simulink model "VCM20_TCon"  (R2021b)
settings: Solver=ode1  StartTime=0.0  StopTime=Inf  FixedStep=0.001  RelTol=1e-3
PostLoadFcn:
  | , if any(exist('dsrtsu_mdlpostloadfcn', 'file') ~= 0), dsrtsu_mdlpostloadfcn('Execute', bdroot); end,
values from neighbouring files (symbols this model uses):
  gear_f = 14.45    [VehicleParamsFEM20_Gear17.m]
  Rwf = 18*(25.4/1000)/2    (= 0.2286)    [VehicleParamsFEM20_Gear17.m]
libraries: rtican x62, dspstat3 x9, simulink x8, rti1401lib_dio_type4 x4, rti1401lib_adc_type4 x4
(part 12 of 12)

== system VCM20_TCon/CAN to EVO4S/relay to EVO4s ==
  from relay board : Inport
  Bus Selector : BusSelector  OutputSignals=AMS_shutdownsig,BSPD_shutdownsig,IMD_shutdownsig
  Data Type Conversion1 : DataTypeConversion
  Data Type Conversion10 : DataTypeConversion
  Data Type Conversion2 : DataTypeConversion
  to EVO4s 704 : rtican/RTICAN Transmit (TX)   Reserved1=[]  Reserved2=[]  Reserved3=[]  Reserved4=[]  SfcnMessage=[]  Msg_Struct=[]  BoardTypeNo=[]  BoardNo=[]  ChannelNo=[]  Parameters=[]  DialogFcn=[]  UnitName=[]  Revision=[]  UnitValues=[]  DSProperties=struct('RTI',struct('Version',uint32(5),'BlockType',struct('isSLSource',uint8(1),'isSLSink',uint8(1),'isHWSource',uint8(0),'isHWSink',uint8(0),'isSetup',uint8(0),'isInline',uint8(1),'isNonInline',uint8(0),'isInterrupt',uint8(0),'isChannelwise',uint8(0)),'IOBoardType','RTICAN','UnitType','MESSAGE','Identifier','TX','DialogType','MSVC','BlockSet','RTICAN','SlaveProcessor','CAN'))  RTIBlockInterface=struct('InputPortsWidth',int32([1 1 1]),'InputPortsActive',[1 1 1],'InputPortsName',{{'AMS_shutdownsig','BSPD_shutdownsig','IMD_shutdownsig'}},'InputPortsDataType',{{'SS_DOUBLE','SS_DOUBLE','SS_DOUBLE'}},'OutputPortsWidth',int32(0),'OutputPortsActive',0,'OutputPortsName',{{''}},'DialogFcn','rtican_message_interface_gui','BlockDisplay',{{'','center'}},'IconTransparency','on','InitLevel',3,'BlockName',struct('Token',{{'CAN_TYPE','_TX_M','_C'}},'BlockParam',{{'BoardTypeNo','BoardNo','ChannelNo'}}),'SampleTime',{{-1}},'TriggerPort',{{'none'}},'EnablePort',{{'none'}})  RTIBlockParameters=struct('BoardTypeNo',{{1,'OFF',[]}},'BoardNo',{{1,'ON',[1 16]}},'ChannelNo',{{2,'ON',[1 2]}},'Parameters',{{struct('DataFileSupport',struct('DataFileSelectedMaster',0,'DataFileSelectedLocal',0,'DataFileName',['<no datafile support>|'],'DataFileDate','','SelectedFile',['<no file selected>']),'Options',struct('StatusSelected',0,'TimeSelected',0,'DeltaTimeSelected',0,'DelayTimeSelected',0,'DelayTimeTXCommandSelected',0,'EncodeSetUnusedBitsToOne',0,'EnableMsgLoopback',0,'TriggerPort',struct('Selected',0,'TriggerType',0),'EnablePortSelected',0,'SignalOnPortnameSelected',1,'UserCoding',struct('Selected',0,'InterfaceFile','UserEncodingFile','FcnName','UserEncodeFcn','InportSelected',0,'InportWidth',1,'OutportSelected',0,'OutportWidth',1),'TerminationMsg',struct('Selected',0,'Byte0_7','0'),'InitialMsg',struct('Selected',0,'Byte0_7','0')),'Message',struct('MsgOnBlocknameSelected',0,'MsgName','EVO4s005','MsgIdFormat',0,'MsgId',1796,'MsgLength',8,'NumSignals',3,'SampleTime',-1,'StartTime',struct('Selected',0,'Value',0),'AutoRepeatTime',struct('Selected',0,'Value',0.1),'Timeout',struct('Selected',0,'Value',0.1),'DelayTime',struct('Selected',0,'Value',0.1),'Signal',struct('SgnName',{'AMS_shutdownsig','BSPD_shutdownsig','IMD_shutdownsig'},'SgnStartBit',{0,1,2},'SgnLength',{1,1,1},'SgnType',{0,0,0},'ModeValue',{-1,-1,-1},'DataType',{1,1,1},'ByteLayout',{1,1,1},'Factor',{1,1,1},'Offset',{0,0,0},'SgnComment',{{''},{''},{''}},'SgnUnit',{'','',''},'Min',{0,0,0},'Max',{0,0,0},'SLDataType',{'SS_DOUBLE','SS_DOUBLE','SS_DOUBLE'}),'MsgIdNumFormat',1,'MsgComment',{{''}}),'Version',1.2,'general',struct('isFromLib',0)),'OFF',[]}},'GroupId',{{struct('Group',{{'RTICAN'}},'No',2,'Behavior',{{'NAMECHANGE'}},'BlockType',{{'SINK'}},'NameChangeFlag',0),'OFF',[]}},'SFcnRTICANMessage',{{struct('MsgType','TX','SFcnPortType','Scalar','MsgName','EVO4s005','MsgIdFormat','STD','MsgId',1796,'MsgLength',8,'NumSignals',3,'SampleTime',-1,'StartTime',struct('Selected','no','Value',0),'AutoRepeatTime',struct('Selected','no','Value',0.1),'Timeout',struct('Selected','no','Value',0.1),'Signal',struct('SgnName',{'AMS_shutdownsig','BSPD_shutdownsig','IMD_shutdownsig'},'SgnStartBit',{0,1,2},'SgnLength',{1,1,1},'SgnType',{'standard','standard','standard'},'ModeValue',{-1,-1,-1},'DataType',{['signed int'],['signed int'],['signed int']},'ByteLayout',{['big endian'],['big endian'],['big endian']},'Factor',{1,1,1},'Offset',{0,0,0},'SLDataType',{'SS_DOUBLE','SS_DOUBLE','SS_DOUBLE'}),'StatusSelected','no','TimeSelected','no','DeltaTimeSelected','no','DelayTimeSelected','no','DelayTimeTXCommandSelected','no','EncodeSetUnusedBitsToOne','no','EnableMsgLoopback','no','TriggerPort',struct('Selected','no','TriggerType',0),'EnablePortSelected','no','UserCoding',struct('Selected','no','InterfaceFile','UserEncodingFile','FcnName','UserEncodeFcn','InportSelected','no','InportWidth',1,'OutportSelected','no','OutportWidth',1),'TerminationMsg',struct('Selected','no','Byte0','0x00','Byte1','0x00','Byte2','0x00','Byte3','0x00','Byte4','0x00','Byte5','0x00','Byte6','0x00','Byte7','0x00'),'InitialMsg',struct('Selected','no','Byte0','0x00','Byte1','0x00','Byte2','0x00','Byte3','0x00','Byte4','0x00','Byte5','0x00','Byte6','0x00','Byte7','0x00'),'BoardType','DS1','BoardNo',1,'ControllerNo',2),'OFF',[]}},'TLCFileName',{{'rtican_tx_message','OFF',[]}})  RTISFcnParameters=struct('SFcnRTICANMessage','struct','TLCFileName','char')  RTIBlockParaDefault=struct('BoardTypeNo',4302,'BoardNo',1,'ChannelNo',1,'Parameters',struct('DataFileSupport',struct('DataFileSelectedMaster',0,'DataFileSelectedLocal',0,'DataFileName','','DataFileDate','','SelectedFile',['<no file selected>']),'Options',struct('StatusSelected',1,'TimeSelected',1,'DeltaTimeSelected',1,'DelayTimeSelected',1,'DelayTimeTXCommandSelected',0,'EncodeSetUnusedBitsToOne',0,'EnableMsgLoopback',0,'TriggerPort',struct('Selected',0,'TriggerType','rising'),'EnablePortSelected',0,'SignalOnPortnameSelected',1,'UserCoding',struct('Selected',0,'InterfaceFile','UserEncodingFile','FcnName','UserEncodeFcn','InportSelected',0,'InportWidth',1,'OutportSelected',0,'OutportWidth',1),'TerminationMsg',struct('Selected',0,'Byte0_7','0'),'InitialMsg',struct('Selected',0,'Byte0_7','0')),'Message',struct('MsgOnBlocknameSelected',0,'MsgName',['TX Message'],'MsgIdFormat',0,'MsgId',100,'MsgLength',8,'NumSignals',1,'SampleTime',-1,'StartTime',struct('Selected',0,'Value',0),'AutoRepeatTime',struct('Selected',0,'Value',0.1),'Timeout',struct('Selected',0,'Value',0.1),'DelayTime',struct('Selected',0,'Value',0.1),'Signal',struct('SgnName',['TX signal'],'SgnStartBit',0,'SgnLength',8,'SgnType',0,'ModeValue',-1,'DataType',0,'SLDataType','SS_DOUBLE','ByteLayout',0,'Factor',1,'Offset',0,'Min',0,'Max',255,'SgnComment',{{}},'SgnUnit',''),'MsgIdNumFormat',0,'MsgComment',{{''}}),'Version',1.2,'general',struct('isFromLib',1)),'GroupId',struct('Group',{{'RTICAN'}},'No',1,'Behavior',{{'NAMECHANGE'}},'BlockType',{{'SINK'}},'NameChangeFlag',0),'SFcnRTICANMessage',struct('MsgType','TX','MsgName',['TX Message'],'MsgIdFormat','STD','MsgId',100,'MsgLength',2,'NumSignals',1,'SampleTime',-1,'StartTime',struct('Selected','no','Value',0),'AutoRepeatTime',struct('Selected','no','Value',0.1),'Timeout',struct('Selected','no','Value',0.1),'DelayTime',struct('Selected','no','Value',0.1),'Signal',struct('SgnName',['TX signal'],'SgnStartBit',0,'SgnLength',8,'SgnType','standard','ModeValue',-1,'DataType',['unsigned int'],'ByteLayout',['little endian'],'SLDataType','SS_DOUBLE','Factor',1,'Offset',0),'StatusSelected','yes','TimeSelected','yes','DeltaTimeSelected','yes','DelayTimeSelected','yes','EnablePortSelected','no','EnableMsgLoopback','no','DelayTimeTXCommandSelected','no','EncodeSetUnusedBitsToOne','no','UserCoding',struct('Selected','no','InterfaceFile','UserDecodingFile','FcnName','UserDecodeFcn','InportSelected','no','InportWidth',1,'OutportSelected','no','OutportWidth',1),'TerminationMsg',struct('Selected','no','Byte0','0x00','Byte1','0x00','Byte2','0x00','Byte3','0x00','Byte4','0x00','Byte5','0x00','Byte6','0x00','Byte7','0x00'),'InitialMsg',struct('Selected','no','Byte0','0x00','Byte1','0x00','Byte2','0x00','Byte3','0x00','Byte4','0x00','Byte5','0x00','Byte6','0x00','Byte7','0x00'),'TriggerPort',struct('Selected','no','TriggerType','rising'),'BoardType','DS4302','BoardNo',1,'ControllerNo',1,'SFcnPortType','Scalar'),'TLCFileName','rtican_tx_message')
      settings: AttributesFormatString=Group Id: RTICAN2\n  SourceProductName=dSPACE RTI CAN Blockset
  wires:
  from relay board/1 -> Bus Selector/1
  Bus Selector/1 -> Data Type Conversion10/1  "<AMS_shutdownsig>"
  Bus Selector/2 -> Data Type Conversion1/1  "<BSPD_shutdownsig>"
  Bus Selector/3 -> Data Type Conversion2/1  "<IMD_shutdownsig>"
  Data Type Conversion10/1 -> to EVO4s 704/1
  Data Type Conversion1/1 -> to EVO4s 704/2
  Data Type Conversion2/1 -> to EVO4s 704/3

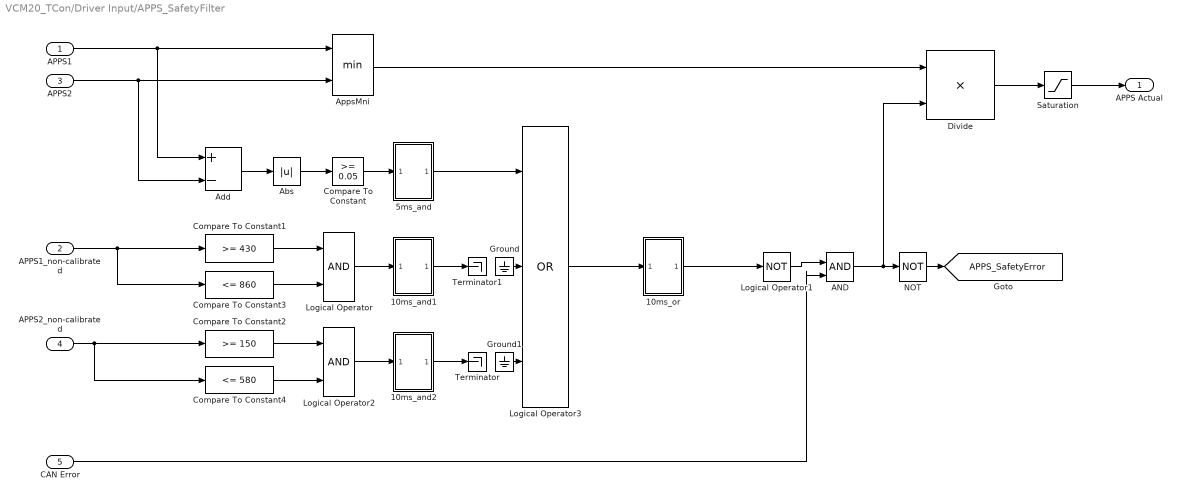
== system VCM20_TCon/Driver Input/APPS_SafetyFilter ==
  APPS1 : Inport
  APPS1_non-calibrated : Inport  Port=2
  APPS2 : Inport  Port=3
  APPS2_non-calibrated : Inport  Port=4
  CAN Error : Inport  Port=5
  10ms_and1 : Subsystem
  10ms_and2 : Subsystem
  10ms_or : Subsystem
  5ms_and : Subsystem
  AND : Logic  IconShape=distinctive  AllPortsSameDT=off  OutDataTypeStr=boolean
  Abs : Abs
  Add : Sum  Inputs=+-
  AppsMni : MinMax  Inputs=2
  Compare To Constant : simulink/Logic and Bit Operations/Compare To Constant  relop=>=  const=0.05  OutDataTypeStr=boolean
  Compare To Constant1 : simulink/Logic and Bit Operations/Compare To Constant  relop=>=  const=430  OutDataTypeStr=boolean
  Compare To Constant2 : simulink/Logic and Bit Operations/Compare To Constant  relop=>=  const=150  OutDataTypeStr=boolean
  Compare To Constant3 : simulink/Logic and Bit Operations/Compare To Constant  relop=<=  const=860  OutDataTypeStr=boolean
  Compare To Constant4 : simulink/Logic and Bit Operations/Compare To Constant  relop=<=  const=580  OutDataTypeStr=boolean
  Divide : Product  Inputs=**
  Ground : Ground
  Ground1 : Ground
  Logical Operator : Logic  AllPortsSameDT=off  OutDataTypeStr=boolean
  Logical Operator1 : Logic  Operator=NOT  AllPortsSameDT=off  OutDataTypeStr=boolean
  Logical Operator2 : Logic  AllPortsSameDT=off  OutDataTypeStr=boolean
  Logical Operator3 : Logic  Operator=OR  Inputs=3  AllPortsSameDT=off  OutDataTypeStr=boolean
  NOT : Logic  Operator=NOT  IconShape=distinctive  AllPortsSameDT=off  OutDataTypeStr=boolean
  Saturation : Saturate  UpperLimit=1  LowerLimit=0
  Terminator : Terminator
  Terminator1 : Terminator
  APPS Actual : Outport  VectorParamsAs1DForOutWhenUnconnected=off
  tag scope: APPS_SafetyError=global
  wires:
  Abs/1 -> Compare To Constant/1
  Add/1 -> Abs/1
  AND/1 -> Divide/2, NOT/1
  Divide/1 -> Saturation/1
  AppsMni/1 -> Divide/1
  Saturation/1 -> APPS Actual/1
  APPS1/1 -> Add/1, AppsMni/1
  APPS2/1 -> Add/2, AppsMni/2
  Compare To Constant/1 -> 5ms_and/1(In1)
  5ms_and/1(Out1) -> Logical Operator3/1
  Compare To Constant3/1 -> Logical Operator/2
  APPS1_non-calibrated/1 -> Compare To Constant3/1, Compare To Constant1/1
  Compare To Constant1/1 -> Logical Operator/1
  Logical Operator/1 -> 10ms_and1/1(In1)
  Compare To Constant4/1 -> Logical Operator2/2
  Compare To Constant2/1 -> Logical Operator2/1
  Logical Operator2/1 -> 10ms_and2/1(In1)
  APPS2_non-calibrated/1 -> Compare To Constant4/1, Compare To Constant2/1
  10ms_and1/1(Out1) -> Terminator1/1
  10ms_and2/1(Out1) -> Terminator/1
  Logical Operator3/1 -> 10ms_or/1(In1)
  Ground/1 -> Logical Operator3/2
  Ground1/1 -> Logical Operator3/3
  CAN Error/1 -> AND/2
  10ms_or/1(Out1) -> Logical Operator1/1
  Logical Operator1/1 -> AND/1
  NOT/1 -> [APPS_SafetyError]

== system VCM20_TCon/Driver Input/Calibration1 ==
  note: キャリブレーション時
      | アクセルを踏んでいないときのAPPS value1の値を上に，
      | アクセル全開のときのAPPS value1の値を下に入れてね．
      | 小数点第3位まで
      |
      | 19/0416記
      | 値のＭＡＸ，ＭＩＮではないよ！
      | そのうち変えますが．
  APPS1_signal : Inport
  APPS1_Scope : Subsystem
  APPS1_signal_lowpass : Scope
  Divide : Product  Inputs=*/  RndMeth=Zero  SaturateOnIntegerOverflow=on
  Moving Average : dspstat3/Moving Average  Method=Sliding window  ForgettingFactorPort=off  SpecifyWindowLength=on  WindowLength=1000  ForgettingFactor=0.9  SimulateUsing=Code generation
  Sum1 : Sum  Inputs=|+-
  Sum3 : Sum  Inputs=-+
  Throttle1_MAX : Constant  Value=517  OutDataTypeStr=double
  Throttle1_MIN : Constant  Value=180  OutDataTypeStr=double
  Transfer Fcn : TransferFcn  Commented=on  Denominator=[1/(2*pi*5) 1]
  APPS1 : Outport  VectorParamsAs1DForOutWhenUnconnected=off
  wires:
  Throttle1_MIN/1 -> Sum1/2, Sum3/1
  Sum3/1 -> Divide/2
  Sum1/1 -> Divide/1
  Throttle1_MAX/1 -> Sum3/2
  Divide/1 -> APPS1/1
  APPS1_signal/1 -> Moving Average/1, Sum1/1, APPS1_Scope/1(APPS1_signal)
  Moving Average/1 -> APPS1_signal_lowpass/1

== system VCM20_TCon/Driver Input/Calibration2 ==
  note: キャリブレーション時
      | アクセルを踏んでいないときのAPPS value２の値を上に，
      | アクセル全開のときのAPPS value２の値を下に入れてね．
      | 小数点第3位まで
      |
      | 19/0416記
      | 値のＭＡＸ，ＭＩＮではないよ！
      | そのうち変えますが．
  APPS2_signal : Inport
  APPS2_Scope : Subsystem
  APPS2_signal_lowpass : Scope
  Divide : Product  Inputs=*/  RndMeth=Zero  SaturateOnIntegerOverflow=on
  Moving Average : dspstat3/Moving Average  Method=Sliding window  ForgettingFactorPort=off  SpecifyWindowLength=on  WindowLength=1000  ForgettingFactor=0.9  SimulateUsing=Code generation
  Sum1 : Sum  Inputs=|+-
  Sum3 : Sum  Inputs=-+
  Throttle2_MAX : Constant  Value=484  OutDataTypeStr=double
  Throttle2_MIN : Constant  Value=829  OutDataTypeStr=double
  Transfer Fcn : TransferFcn  Commented=on  Denominator=[1/(2*pi*5) 1]
  APPS2 : Outport  VectorParamsAs1DForOutWhenUnconnected=off
  wires:
  Throttle2_MIN/1 -> Sum3/1, Sum1/2
  Sum3/1 -> Divide/2
  Sum1/1 -> Divide/1
  Throttle2_MAX/1 -> Sum3/2
  Divide/1 -> APPS2/1
  APPS2_signal/1 -> Moving Average/1, Sum1/1, APPS2_Scope/1(In1)
  Moving Average/1 -> APPS2_signal_lowpass/1

== system VCM20_TCon/Driver Input/Calibration3 ==
  note: 左全切り
  note: 反時計回りが正
      | 時計回りが負
  note: 右全切り
  SWAS1_signal : Inport
  Add : Sum  Inputs=+-
  Add1 : Sum  Inputs=+-
  Add2 : Sum  Inputs=-+
  Divide : Product  Inputs=/*
  Divide1 : Product  Inputs=*/
  Gain1 : Gain  Gain=-1
  LeftMax_deg : Gain  Gain=95
  Moving Average : dspstat3/Moving Average  Method=Sliding window  ForgettingFactorPort=off  SpecifyWindowLength=on  WindowLength=1000  ForgettingFactor=0.9  SimulateUsing=Code generation
  RightMax_deg : Gain  Gain=85
  SWAS1_MovingAverage : Scope
  SWAS1_signal_0deg : Constant  Value=0.279
  SWAS1_signal_minus : Constant  Value=0.403
  SWAS1_signal_plus : Constant  Value=0.148
  Switch : Switch  Criteria=u2 > Threshold
  Transfer Fcn : TransferFcn  Denominator=[1/(2*pi*5) 1]
  SWAS1 : Outport  VectorParamsAs1DForOutWhenUnconnected=off
  wires:
  SWAS1_signal/1 -> Transfer Fcn/1
  SWAS1_signal_0deg/1 -> Add2/1, Add1/2, Add/2
  Add/1 -> Divide1/1, Divide/2, Switch/2
  SWAS1_signal_plus/1 -> Add1/1
  Add1/1 -> Divide/1
  Divide/1 -> LeftMax_deg/1
  LeftMax_deg/1 -> Switch/1
  SWAS1_signal_minus/1 -> Add2/2
  Add2/1 -> Divide1/2
  Divide1/1 -> Gain1/1
  Gain1/1 -> RightMax_deg/1
  Switch/1 -> SWAS1/1
  Transfer Fcn/1 -> Moving Average/1, Add/1
  Moving Average/1 -> SWAS1_MovingAverage/1
  RightMax_deg/1 -> Switch/3

== system VCM20_TCon/Driver Input/Calibration4 ==
  note: 左全切り
  note: 反時計回りが正
      | 時計回りが負
  note: 右全切り
  SWAS2_signal : Inport
  Add : Sum  Inputs=+-
  Add1 : Sum  Inputs=+-
  Add2 : Sum  Inputs=-+
  Divide : Product  Inputs=/*
  Divide1 : Product  Inputs=*/
  Gain1 : Gain  Gain=-1
  LeftMax_deg : Gain  Gain=85
  Moving Average : dspstat3/Moving Average  Method=Sliding window  ForgettingFactorPort=off  SpecifyWindowLength=on  WindowLength=1000  ForgettingFactor=0.9  SimulateUsing=Code generation
  RightMax_deg : Gain  Gain=95
  SWAS2_MovingAverage : Scope
  SWAS2_signal_0deg : Constant  Value=520
  SWAS2_signal_minus : Constant  Value=252
  SWAS2_signal_plus : Constant  Value=789
  Switch : Switch  Criteria=u2 > Threshold
  Transfer Fcn : TransferFcn  Denominator=[1/(2*pi*5) 1]
  SWAS2 : Outport  VectorParamsAs1DForOutWhenUnconnected=off
  wires:
  LeftMax_deg/1 -> Switch/3
  Moving Average/1 -> SWAS2_MovingAverage/1
  Switch/1 -> SWAS2/1
  Divide1/1 -> LeftMax_deg/1
  Add2/1 -> Divide1/2
  RightMax_deg/1 -> Switch/1
  Divide/1 -> Gain1/1
  Add1/1 -> Divide/1
  Add/1 -> Switch/2, Divide/2, Divide1/1
  SWAS2_signal/1 -> Transfer Fcn/1
  Transfer Fcn/1 -> Add/1, Moving Average/1
  SWAS2_signal_minus/1 -> Add2/2
  SWAS2_signal_plus/1 -> Add1/1
  SWAS2_signal_0deg/1 -> Add/2, Add1/2, Add2/1
  Gain1/1 -> RightMax_deg/1

== system VCM20_TCon/Driver Input/Calibration5 ==
  BrakePressF_signal : Inport
  BrakePressF_Pa : Display
  BrakePressF : Outport  VectorParamsAs1DForOutWhenUnconnected=off
  wires:
  BrakePressF_signal/1 -> BrakePressF_Pa/1, BrakePressF/1

== system VCM20_TCon/Driver Input/Calibration6 ==
  BrakePressR_signal : Inport
  BrakePressR_Pa : Display
  BrakePressR : Outport  VectorParamsAs1DForOutWhenUnconnected=off
  wires:
  BrakePressR_signal/1 -> BrakePressR_Pa/1, BrakePressR/1

== system VCM20_TCon/Driver Input/Calibration7 ==
  note: キャリブレーション時
      | アクセルを踏んでいないときのAPPS value1の値を上に，
      | アクセル全開のときのAPPS value1の値を下に入れてね．
      | 小数点第3位まで
      |
      | 19/0416記
      | 値のＭＡＸ，ＭＩＮではないよ！
      | そのうち変えますが．
  BrakePressF_signal : Inport
  BrakePressF_MAX : Constant  Value=515  OutDataTypeStr=double
  BrakePressF_MIN : Constant  Value=826  OutDataTypeStr=double
  BrakePressF_Scope : Subsystem
  BrakePressF_signal_lowpass : Scope
  Divide : Product  Inputs=*/  RndMeth=Zero  SaturateOnIntegerOverflow=on
  Moving Average : dspstat3/Moving Average  Method=Sliding window  ForgettingFactorPort=off  SpecifyWindowLength=on  WindowLength=1000  ForgettingFactor=0.9  SimulateUsing=Code generation
  Sum1 : Sum  Inputs=|+-
  Sum3 : Sum  Inputs=-+
  BrakePressF : Outport  VectorParamsAs1DForOutWhenUnconnected=off
  wires:
  BrakePressF_MIN/1 -> Sum1/2, Sum3/1
  Sum3/1 -> Divide/2
  Sum1/1 -> Divide/1
  BrakePressF_MAX/1 -> Sum3/2
  Divide/1 -> BrakePressF/1
  BrakePressF_signal/1 -> Moving Average/1, Sum1/1, BrakePressF_Scope/1(BrakePressF_signal)
  Moving Average/1 -> BrakePressF_signal_lowpass/1

== system VCM20_TCon/Driver Input/SWAS_SafetyFilter1 ==
  note: 異常時はVDCOffにする
  note: タイヤの切れ角
  SWAS1 : Inport
  SWAS1_non-calibrated : Inport  Port=2
  SWAS2 : Inport  Port=3
  SWAS2_non-calibrated : Inport  Port=4
  CAN Error : Inport  Port=5
  10ms_and1 : Subsystem
  AND : Logic  IconShape=distinctive  AllPortsSameDT=off  OutDataTypeStr=boolean
  Compare To Constant1 : simulink/Logic and Bit Operations/Compare To Constant  relop=>=  const=250  OutDataTypeStr=boolean
  Compare To Constant3 : simulink/Logic and Bit Operations/Compare To Constant  relop=<=  const=791  OutDataTypeStr=boolean
  Divide : Product  Inputs=**
  Logical Operator : Logic  AllPortsSameDT=off  OutDataTypeStr=boolean
  Logical Operator1 : Logic  Operator=NOT  AllPortsSameDT=off  OutDataTypeStr=boolean
  Saturation : Saturate  UpperLimit=180  LowerLimit=-180
  SteerAngle_deg : Gain  Gain=1/5.65
  SteerAngle_rad : Gain  Gain=pi/180
  Terminator1 : Terminator
  Terminator2 : Terminator
  SteerAngle_Actual : Outport  VectorParamsAs1DForOutWhenUnconnected=off
  tag scope: Steer_SafetyError=global
  wires:
  AND/1 -> Divide/2, Logical Operator1/1
  Logical Operator/1 -> 10ms_and1/1(In1)
  Compare To Constant1/1 -> Logical Operator/1
  SWAS2_non-calibrated/1 -> Compare To Constant3/1, Compare To Constant1/1
  Compare To Constant3/1 -> Logical Operator/2
  Saturation/1 -> SteerAngle_deg/1
  SWAS2/1 -> Divide/1
  Logical Operator1/1 -> [Steer_SafetyError]
  Divide/1 -> Saturation/1
  SteerAngle_rad/1 -> SteerAngle_Actual/1
  SteerAngle_deg/1 -> SteerAngle_rad/1
  CAN Error/1 -> AND/2
  10ms_and1/1(Out1) -> AND/1
  SWAS1/1 -> Terminator1/1
  SWAS1_non-calibrated/1 -> Terminator2/1

== system VCM20_TCon/RTI Data/RTI Data Store ==
  RTI Data Store : Subsystem  mask(RTI_DATA_STORE){}
      mask help:
      | RTI Data Store Block. This block is used by RTI to store internal model dependent data. Deleting this block will result in data loss.
      |
      | NEVER DELETE, COPY, OR MODIFY THIS BLOCK!
      mask Help:
      | RTI Data Store Block. This block is used by RTI to store internal model dependent data. Deleting this block will result in data loss.
      | 
      | NEVER DELETE, COPY, OR MODIFY THIS BLOCK!
      mask Display: text(0.5, 0.5, ' ', 'HorizontalAlignment', 'center');

== system VCM20_TCon/sensors from cooling/Subsystem ==
  note: [温度]=-21.188×[電圧]+105.95
      | サーミスタ公正.xlsx参照
  In1 : Inport
  Add : Sum  Inputs=+-
  Constant : Constant  Value=-21.188
  Constant1 : Constant  Value=105.95
  Product : Product
  reikyaku_temp1 : Outport  VectorParamsAs1DForOutWhenUnconnected=off
  wires:
  In1/1 -> Product/2
  Add/1 -> reikyaku_temp1/1  "reikyaku_temp1"
  Product/1 -> Add/1
  Constant1/1 -> Add/2
  Constant/1 -> Product/1

== system VCM20_TCon/sensors from cooling/Subsystem1 ==
  In1 : Inport
  Add : Sum  Inputs=+-
  Constant : Constant  Value=-21.188
  Constant1 : Constant  Value=105.95
  Product : Product
  reikyaku_temp2 : Outport  VectorParamsAs1DForOutWhenUnconnected=off
  wires:
  In1/1 -> Product/2
  Add/1 -> reikyaku_temp2/1  "reikyaku_temp2"
  Product/1 -> Add/1
  Constant1/1 -> Add/2
  Constant/1 -> Product/1

== system VCM20_TCon/sensors from cooling/Subsystem2 ==
  In1 : Inport
  Add : Sum  Inputs=+-
  Constant : Constant  Value=-21.188
  Constant1 : Constant  Value=105.95
  Product : Product
  reikyaku_temp3 : Outport  VectorParamsAs1DForOutWhenUnconnected=off
  wires:
  In1/1 -> Product/2
  Add/1 -> reikyaku_temp3/1  "reikyaku_temp3"
  Product/1 -> Add/1
  Constant1/1 -> Add/2
  Constant/1 -> Product/1

== system VCM20_TCon/speedlimit/kph to motor rpm ==
  kph : Inport
  Gear : Gain  Gain=gear_f
  to m/s : Gain  Gain=1000/3600
  toTire_rpm : Gain  Gain=60/(2*pi*Rwf)
  rpm : Outport  VectorParamsAs1DForOutWhenUnconnected=off
  wires:
  kph/1 -> to m/s/1
  toTire_rpm/1 -> Gear/1
  to m/s/1 -> toTire_rpm/1
  Gear/1 -> rpm/1

== system VCM20_TCon/Driver Input/APPS_SafetyFilter/10ms_and1 ==
  In1 : Inport
  Delay : Delay  DelayLength=0  InitialCondition=0
  Delay1 : Delay  DelayLength=1  InitialCondition=0
  Delay2 : Delay  InitialCondition=0
  Delay3 : Delay  DelayLength=3  InitialCondition=0
  Delay4 : Delay  DelayLength=4  InitialCondition=0
  Delay5 : Delay  DelayLength=5  InitialCondition=0
  Delay6 : Delay  DelayLength=6  InitialCondition=0
  Delay7 : Delay  DelayLength=7  InitialCondition=0
  Delay8 : Delay  DelayLength=8  InitialCondition=0
  Delay9 : Delay  DelayLength=9  InitialCondition=0
  Logical Operator : Logic  Inputs=10  AllPortsSameDT=off  OutDataTypeStr=boolean
  Out1 : Outport  VectorParamsAs1DForOutWhenUnconnected=off
  wires:
  Delay2/1 -> Logical Operator/3
  Delay8/1 -> Logical Operator/9
  In1/1 -> Delay9/1, Delay8/1, Delay7/1, Delay6/1, Delay5/1, Delay4/1, Delay3/1, Delay2/1, Delay1/1, Delay/1
  Delay/1 -> Logical Operator/1
  Delay1/1 -> Logical Operator/2
  Delay3/1 -> Logical Operator/4
  Delay4/1 -> Logical Operator/5
  Delay9/1 -> Logical Operator/10
  Delay5/1 -> Logical Operator/6
  Delay7/1 -> Logical Operator/8
  Delay6/1 -> Logical Operator/7
  Logical Operator/1 -> Out1/1

== system VCM20_TCon/Driver Input/APPS_SafetyFilter/10ms_and2 ==
  In1 : Inport
  Delay : Delay  DelayLength=0  InitialCondition=0
  Delay1 : Delay  DelayLength=1  InitialCondition=0
  Delay2 : Delay  InitialCondition=0
  Delay3 : Delay  DelayLength=3  InitialCondition=0
  Delay4 : Delay  DelayLength=4  InitialCondition=0
  Delay5 : Delay  DelayLength=5  InitialCondition=0
  Delay6 : Delay  DelayLength=6  InitialCondition=0
  Delay7 : Delay  DelayLength=7  InitialCondition=0
  Delay8 : Delay  DelayLength=8  InitialCondition=0
  Delay9 : Delay  DelayLength=9  InitialCondition=0
  Logical Operator : Logic  Inputs=10  AllPortsSameDT=off  OutDataTypeStr=boolean
  Out1 : Outport  VectorParamsAs1DForOutWhenUnconnected=off
  wires:
  Delay2/1 -> Logical Operator/3
  Delay8/1 -> Logical Operator/9
  In1/1 -> Delay9/1, Delay8/1, Delay7/1, Delay6/1, Delay5/1, Delay4/1, Delay3/1, Delay2/1, Delay1/1, Delay/1
  Delay/1 -> Logical Operator/1
  Delay1/1 -> Logical Operator/2
  Delay3/1 -> Logical Operator/4
  Delay4/1 -> Logical Operator/5
  Delay9/1 -> Logical Operator/10
  Delay5/1 -> Logical Operator/6
  Delay7/1 -> Logical Operator/8
  Delay6/1 -> Logical Operator/7
  Logical Operator/1 -> Out1/1

== system VCM20_TCon/Driver Input/APPS_SafetyFilter/10ms_or ==
  In1 : Inport
  Compare To Constant : simulink/Logic and Bit Operations/Compare To Constant  relop=>  const=0  OutDataTypeStr=boolean
  Data Type Conversion : DataTypeConversion  OutDataTypeStr=single
  Delay : Delay  Commented=on  DelayLength=0  InitialCondition=0
  Delay1 : Delay  Commented=on  DelayLength=1  InitialCondition=0
  Delay2 : Delay  Commented=on  InitialCondition=0
  Delay3 : Delay  Commented=on  DelayLength=3  InitialCondition=0
  Delay4 : Delay  Commented=on  DelayLength=4  InitialCondition=0
  Delay5 : Delay  Commented=on  DelayLength=5  InitialCondition=0
  Delay6 : Delay  Commented=on  DelayLength=6  InitialCondition=0
  Delay7 : Delay  Commented=on  DelayLength=7  InitialCondition=0
  Delay8 : Delay  Commented=on  DelayLength=8  InitialCondition=0
  Delay9 : Delay  Commented=on  DelayLength=9  InitialCondition=0
  Logical Operator : Logic  Commented=on  Operator=OR  Inputs=10  AllPortsSameDT=off  OutDataTypeStr=boolean
  Moving Average : dspstat3/Moving Average  Method=Sliding window  ForgettingFactorPort=off  SpecifyWindowLength=on  WindowLength=200  ForgettingFactor=0.9  SimulateUsing=Code generation
  Out1 : Outport  VectorParamsAs1DForOutWhenUnconnected=off
  wires:
  Delay2/1 -> Logical Operator/3
  Delay8/1 -> Logical Operator/9
  In1/1 -> Data Type Conversion/1, Delay9/1, Delay8/1, Delay7/1, Delay6/1, Delay5/1, Delay4/1, Delay3/1, Delay2/1, Delay1/1, Delay/1
  Delay/1 -> Logical Operator/1
  Delay1/1 -> Logical Operator/2
  Delay3/1 -> Logical Operator/4
  Delay4/1 -> Logical Operator/5
  Delay9/1 -> Logical Operator/10
  Delay5/1 -> Logical Operator/6
  Delay7/1 -> Logical Operator/8
  Delay6/1 -> Logical Operator/7
  Logical Operator/1 -> ?
  Moving Average/1 -> Compare To Constant/1
  Compare To Constant/1 -> Out1/1
  Data Type Conversion/1 -> Moving Average/1

== system VCM20_TCon/Driver Input/APPS_SafetyFilter/5ms_and ==
  In1 : Inport
  Delay : Delay  DelayLength=0  InitialCondition=0
  Delay1 : Delay  DelayLength=1  InitialCondition=0
  Delay2 : Delay  InitialCondition=0
  Delay3 : Delay  DelayLength=3  InitialCondition=0
  Delay4 : Delay  DelayLength=4  InitialCondition=0
  Logical Operator : Logic  Inputs=5  AllPortsSameDT=off  OutDataTypeStr=boolean
  Out1 : Outport  VectorParamsAs1DForOutWhenUnconnected=off
  wires:
  Delay2/1 -> Logical Operator/3
  In1/1 -> Delay4/1, Delay3/1, Delay2/1, Delay1/1, Delay/1
  Delay/1 -> Logical Operator/1
  Delay1/1 -> Logical Operator/2
  Delay3/1 -> Logical Operator/4
  Delay4/1 -> Logical Operator/5
  Logical Operator/1 -> Out1/1

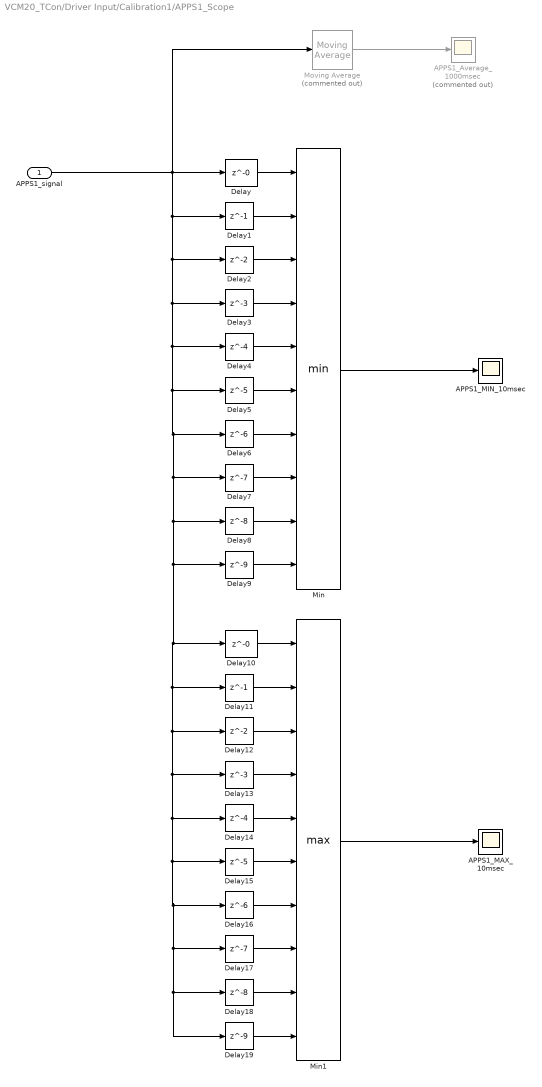
== system VCM20_TCon/Driver Input/Calibration1/APPS1_Scope ==
  APPS1_signal : Inport
  APPS1_Average_1000msec : Scope  Commented=on
  APPS1_MAX_10msec : Scope
  APPS1_MIN_10msec : Scope
  Delay : Delay  DelayLength=0  InitialCondition=0
  Delay1 : Delay  DelayLength=1  InitialCondition=0
  Delay10 : Delay  DelayLength=0  InitialCondition=0
  Delay11 : Delay  DelayLength=1  InitialCondition=0
  Delay12 : Delay  InitialCondition=0
  Delay13 : Delay  DelayLength=3  InitialCondition=0
  Delay14 : Delay  DelayLength=4  InitialCondition=0
  Delay15 : Delay  DelayLength=5  InitialCondition=0
  Delay16 : Delay  DelayLength=6  InitialCondition=0
  Delay17 : Delay  DelayLength=7  InitialCondition=0
  Delay18 : Delay  DelayLength=8  InitialCondition=0
  Delay19 : Delay  DelayLength=9  InitialCondition=0
  Delay2 : Delay  InitialCondition=0
  Delay3 : Delay  DelayLength=3  InitialCondition=0
  Delay4 : Delay  DelayLength=4  InitialCondition=0
  Delay5 : Delay  DelayLength=5  InitialCondition=0
  Delay6 : Delay  DelayLength=6  InitialCondition=0
  Delay7 : Delay  DelayLength=7  InitialCondition=0
  Delay8 : Delay  DelayLength=8  InitialCondition=0
  Delay9 : Delay  DelayLength=9  InitialCondition=0
  Min : MinMax  Inputs=10
  Min1 : MinMax  Function=max  Inputs=10
  Moving Average : dspstat3/Moving Average  Commented=on  Method=Sliding window  ForgettingFactorPort=off  SpecifyWindowLength=on  WindowLength=1000  ForgettingFactor=0.9  SimulateUsing=Code generation
  wires:
  Min/1 -> APPS1_MIN_10msec/1
  Delay5/1 -> Min/6
  Delay2/1 -> Min/3
  Delay9/1 -> Min/10
  Delay/1 -> Min/1
  Delay8/1 -> Min/9
  Delay1/1 -> Min/2
  Delay3/1 -> Min/4
  Delay4/1 -> Min/5
  Delay7/1 -> Min/8
  Delay6/1 -> Min/7
  Delay13/1 -> Min1/4
  Delay18/1 -> Min1/9
  Delay14/1 -> Min1/5
  Delay10/1 -> Min1/1
  Delay19/1 -> Min1/10
  Delay15/1 -> Min1/6
  Delay16/1 -> Min1/7
  Delay17/1 -> Min1/8
  Delay11/1 -> Min1/2
  Delay12/1 -> Min1/3
  Min1/1 -> APPS1_MAX_10msec/1
  Moving Average/1 -> APPS1_Average_1000msec/1
  APPS1_signal/1 -> Moving Average/1, Delay1/1, Delay2/1, Delay3/1, Delay5/1, Delay6/1, Delay8/1, Delay11/1, Delay12/1, Delay13/1, Delay15/1, Delay16/1, Delay18/1, Delay19/1, Delay17/1, Delay14/1, Delay10/1, Delay9/1, Delay7/1, Delay4/1, Delay/1

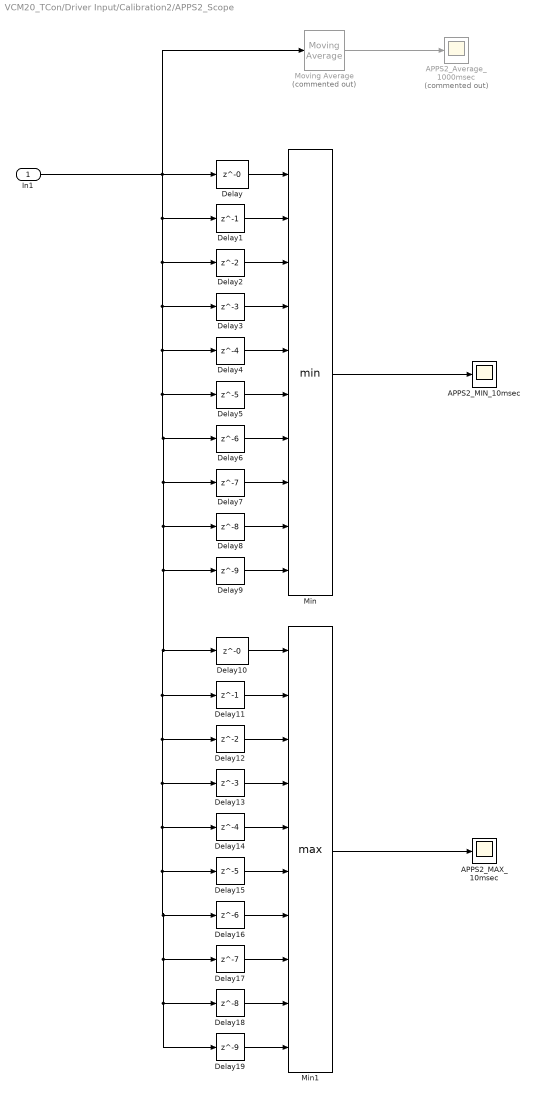
== system VCM20_TCon/Driver Input/Calibration2/APPS2_Scope ==
  In1 : Inport
  APPS2_Average_1000msec : Scope  Commented=on
  APPS2_MAX_10msec : Scope
  APPS2_MIN_10msec : Scope
  Delay : Delay  DelayLength=0  InitialCondition=0
  Delay1 : Delay  DelayLength=1  InitialCondition=0
  Delay10 : Delay  DelayLength=0  InitialCondition=0
  Delay11 : Delay  DelayLength=1  InitialCondition=0
  Delay12 : Delay  InitialCondition=0
  Delay13 : Delay  DelayLength=3  InitialCondition=0
  Delay14 : Delay  DelayLength=4  InitialCondition=0
  Delay15 : Delay  DelayLength=5  InitialCondition=0
  Delay16 : Delay  DelayLength=6  InitialCondition=0
  Delay17 : Delay  DelayLength=7  InitialCondition=0
  Delay18 : Delay  DelayLength=8  InitialCondition=0
  Delay19 : Delay  DelayLength=9  InitialCondition=0
  Delay2 : Delay  InitialCondition=0
  Delay3 : Delay  DelayLength=3  InitialCondition=0
  Delay4 : Delay  DelayLength=4  InitialCondition=0
  Delay5 : Delay  DelayLength=5  InitialCondition=0
  Delay6 : Delay  DelayLength=6  InitialCondition=0
  Delay7 : Delay  DelayLength=7  InitialCondition=0
  Delay8 : Delay  DelayLength=8  InitialCondition=0
  Delay9 : Delay  DelayLength=9  InitialCondition=0
  Min : MinMax  Inputs=10
  Min1 : MinMax  Function=max  Inputs=10
  Moving Average : dspstat3/Moving Average  Commented=on  Method=Sliding window  ForgettingFactorPort=off  SpecifyWindowLength=on  WindowLength=1000  ForgettingFactor=0.9  SimulateUsing=Code generation
  wires:
  Min/1 -> APPS2_MIN_10msec/1
  Delay5/1 -> Min/6
  Delay2/1 -> Min/3
  Delay9/1 -> Min/10
  Delay/1 -> Min/1
  Delay8/1 -> Min/9
  Delay1/1 -> Min/2
  Delay3/1 -> Min/4
  Delay4/1 -> Min/5
  Delay7/1 -> Min/8
  Delay6/1 -> Min/7
  Delay13/1 -> Min1/4
  Delay18/1 -> Min1/9
  Delay14/1 -> Min1/5
  Delay10/1 -> Min1/1
  Delay19/1 -> Min1/10
  Delay15/1 -> Min1/6
  Delay16/1 -> Min1/7
  Delay17/1 -> Min1/8
  Delay11/1 -> Min1/2
  Delay12/1 -> Min1/3
  Min1/1 -> APPS2_MAX_10msec/1
  In1/1 -> Moving Average/1, Delay1/1, Delay2/1, Delay3/1, Delay5/1, Delay6/1, Delay8/1, Delay11/1, Delay12/1, Delay13/1, Delay15/1, Delay16/1, Delay18/1, Delay19/1, Delay17/1, Delay14/1, Delay10/1, Delay9/1, Delay7/1, Delay4/1, Delay/1
  Moving Average/1 -> APPS2_Average_1000msec/1

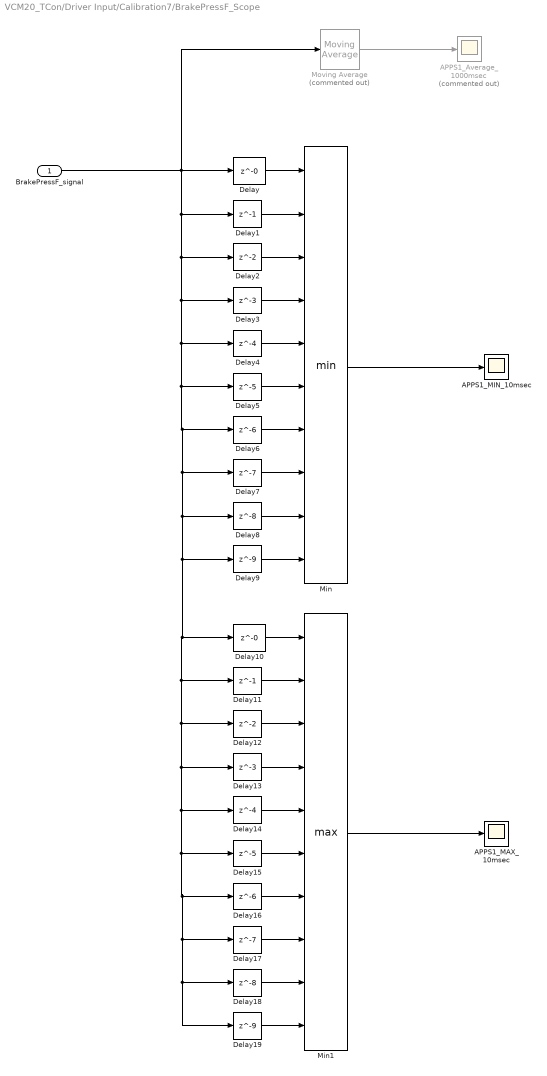
== system VCM20_TCon/Driver Input/Calibration7/BrakePressF_Scope ==
  BrakePressF_signal : Inport
  APPS1_Average_1000msec : Scope  Commented=on
  APPS1_MAX_10msec : Scope
  APPS1_MIN_10msec : Scope
  Delay : Delay  DelayLength=0  InitialCondition=0
  Delay1 : Delay  DelayLength=1  InitialCondition=0
  Delay10 : Delay  DelayLength=0  InitialCondition=0
  Delay11 : Delay  DelayLength=1  InitialCondition=0
  Delay12 : Delay  InitialCondition=0
  Delay13 : Delay  DelayLength=3  InitialCondition=0
  Delay14 : Delay  DelayLength=4  InitialCondition=0
  Delay15 : Delay  DelayLength=5  InitialCondition=0
  Delay16 : Delay  DelayLength=6  InitialCondition=0
  Delay17 : Delay  DelayLength=7  InitialCondition=0
  Delay18 : Delay  DelayLength=8  InitialCondition=0
  Delay19 : Delay  DelayLength=9  InitialCondition=0
  Delay2 : Delay  InitialCondition=0
  Delay3 : Delay  DelayLength=3  InitialCondition=0
  Delay4 : Delay  DelayLength=4  InitialCondition=0
  Delay5 : Delay  DelayLength=5  InitialCondition=0
  Delay6 : Delay  DelayLength=6  InitialCondition=0
  Delay7 : Delay  DelayLength=7  InitialCondition=0
  Delay8 : Delay  DelayLength=8  InitialCondition=0
  Delay9 : Delay  DelayLength=9  InitialCondition=0
  Min : MinMax  Inputs=10
  Min1 : MinMax  Function=max  Inputs=10
  Moving Average : dspstat3/Moving Average  Commented=on  Method=Sliding window  ForgettingFactorPort=off  SpecifyWindowLength=on  WindowLength=1000  ForgettingFactor=0.9  SimulateUsing=Code generation
  wires:
  Min/1 -> APPS1_MIN_10msec/1
  Delay5/1 -> Min/6
  Delay2/1 -> Min/3
  Delay9/1 -> Min/10
  Delay/1 -> Min/1
  Delay8/1 -> Min/9
  Delay1/1 -> Min/2
  Delay3/1 -> Min/4
  Delay4/1 -> Min/5
  Delay7/1 -> Min/8
  Delay6/1 -> Min/7
  Delay13/1 -> Min1/4
  Delay18/1 -> Min1/9
  Delay14/1 -> Min1/5
  Delay10/1 -> Min1/1
  Delay19/1 -> Min1/10
  Delay15/1 -> Min1/6
  Delay16/1 -> Min1/7
  Delay17/1 -> Min1/8
  Delay11/1 -> Min1/2
  Delay12/1 -> Min1/3
  Min1/1 -> APPS1_MAX_10msec/1
  Moving Average/1 -> APPS1_Average_1000msec/1
  BrakePressF_signal/1 -> Moving Average/1, Delay1/1, Delay2/1, Delay3/1, Delay5/1, Delay6/1, Delay8/1, Delay11/1, Delay12/1, Delay13/1, Delay15/1, Delay16/1, Delay18/1, Delay19/1, Delay17/1, Delay14/1, Delay10/1, Delay9/1, Delay7/1, Delay4/1, Delay/1

== system VCM20_TCon/Driver Input/SWAS_SafetyFilter1/10ms_and1 ==
  In1 : Inport
  Delay : Delay  DelayLength=0  InitialCondition=0
  Delay1 : Delay  DelayLength=1  InitialCondition=0
  Delay2 : Delay  InitialCondition=0
  Delay3 : Delay  DelayLength=3  InitialCondition=0
  Delay4 : Delay  DelayLength=4  InitialCondition=0
  Delay5 : Delay  DelayLength=5  InitialCondition=0
  Delay6 : Delay  DelayLength=6  InitialCondition=0
  Delay7 : Delay  DelayLength=7  InitialCondition=0
  Delay8 : Delay  DelayLength=8  InitialCondition=0
  Delay9 : Delay  DelayLength=9  InitialCondition=0
  Logical Operator : Logic  Inputs=10  AllPortsSameDT=off  OutDataTypeStr=boolean
  Out1 : Outport  VectorParamsAs1DForOutWhenUnconnected=off
  wires:
  Logical Operator/1 -> Out1/1
  Delay6/1 -> Logical Operator/7
  Delay7/1 -> Logical Operator/8
  Delay5/1 -> Logical Operator/6
  Delay9/1 -> Logical Operator/10
  Delay4/1 -> Logical Operator/5
  Delay3/1 -> Logical Operator/4
  Delay1/1 -> Logical Operator/2
  Delay/1 -> Logical Operator/1
  In1/1 -> Delay/1, Delay1/1, Delay2/1, Delay3/1, Delay4/1, Delay5/1, Delay6/1, Delay7/1, Delay8/1, Delay9/1
  Delay8/1 -> Logical Operator/9
  Delay2/1 -> Logical Operator/3

== system VCM20_TCon/RTI Data/RTI Data Store/RTI Data Store ==
  RTI Data Store : Subsystem  mask(RTI_DATA_STORE){}
      mask help:
      | RTI Data Store Block. This block is used by RTI to store internal model dependent data. Deleting this block will result in data loss.
      |
      | NEVER DELETE, COPY, OR MODIFY THIS BLOCK!
      mask Help:
      | RTI Data Store Block. This block is used by RTI to store internal model dependent data. Deleting this block will result in data loss.
      | 
      | NEVER DELETE, COPY, OR MODIFY THIS BLOCK!
      mask Display: text(0.5, 0.5, ' ', 'HorizontalAlignment', 'center');

== system VCM20_TCon/RTI Data/RTI Data Store/RTI Data Store/RTI Data Store ==
  RTI Data Store : Subsystem  mask(RTI_DATA_STORE){}
      mask help:
      | RTI Data Store Block. This block is used by RTI to store internal model dependent data. Deleting this block will result in data loss.
      |
      | NEVER DELETE, COPY, OR MODIFY THIS BLOCK!
      mask Help:
      | RTI Data Store Block. This block is used by RTI to store internal model dependent data. Deleting this block will result in data loss.
      | 
      | NEVER DELETE, COPY, OR MODIFY THIS BLOCK!
      mask Display: text(0.5, 0.5, ' ', 'HorizontalAlignment', 'center');

== system VCM20_TCon/RTI Data/RTI Data Store/RTI Data Store/RTI Data Store/RTI Data Store ==

== stateflow chart VCM20_TCon/VCMOutput/Steer Chart ==
  state Gain2
    entry:
    LCDtext = uint8('Gain2   ');
    LCDnumber = gain2;
  state Start
    entry:
    gain1 = 5;
    gain1max = 20;
    gain1min = 0;
    gain2 = 10;
    gain2max = 15;
    gain2min = 5;
  state Display1
    entry:
    LCDtext = uint8('IMUStat ');
    LCDnumber = Display1number;
  state Gain1
    entry:
    LCDtext = uint8('Gain1   ');
    LCDnumber = gain1;
  state Select3
  state Select1
  state Select2
  state Plus_Gain2
    entry:
    gain2 = gain2 + 1;
    LCDnumber = gain2;
  state Minus_Gain2
    entry:
    gain2 = gain2 - 1;
    LCDnumber = gain2;
  state Plus_Gain1
    entry:
    gain1 = gain1 + 1;
    LCDnumber = gain1;
  state Minus_Gain1
    entry:
    gain1 = gain1 - 1;
    LCDnumber = gain1;
  Select3 -> Display1 : [SelectSW == 0]
  (default) -> Start
  Start -> Display1
  Gain2 -> Select3 [order 3] : [SelectSW == 1]
  Display1 -> Select1 : [SelectSW == 1]
  Gain1 -> Select2 [order 3] : [SelectSW == 1]
  Select2 -> Gain2 : [SelectSW == 0]
  Select1 -> Gain1 : [SelectSW == 0]
  Gain2 -> Plus_Gain2 [order 1] : [PlusSW == 1 & gain2 < gain2max]
  Plus_Gain2 -> Gain2 : [PlusSW == 0]
  Gain2 -> Minus_Gain2 [order 2] : [MinusSW == 1 & gain2 > gain2min]
  Minus_Gain2 -> Gain2 : [MinusSW == 0]
  Gain1 -> Plus_Gain1 [order 1] : [PlusSW == 1 & gain1 < gain1max]
  Plus_Gain1 -> Gain1 : [PlusSW == 0]
  Gain1 -> Minus_Gain1 [order 2] : [MinusSW == 1 & gain1 > gain1min]
  Minus_Gain1 -> Gain1 : [MinusSW == 0]
  data: MinusSW input; PlusSW input; SelectSW input; LCDnumber output; LCDtext output; gain1max local; gain1min local; gain2max local; gain2min local; Display1number input; gain1 output; gain2 output
